simulink model "digitalIntegration"  (R2020a)
settings: Solver=FixedStepDiscrete  StartTime=0.0  StopTime=20  FixedStep=T  RelTol=1e-3
undefined symbols (not defined in the file): T
settings Model: Creator=mtcer  LastModifiedBy=mc218k
settings DataIOCC: ReturnWorkspaceOutputs=off
settings DebuggingCC: ArithmeticOperatorsInVariantConditions=warning
settings SFSimCC: CustomCodeUndefinedFunction=UseInterfaceOnly

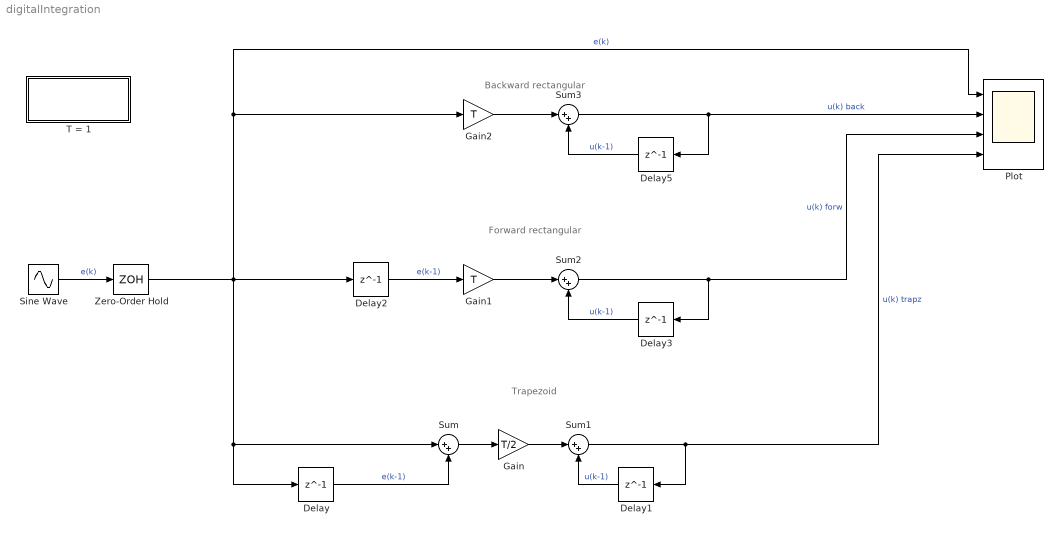
== system digitalIntegration ==
  note: Forward rectangular
  note: Trapezoid
  note: Backward rectangular
  Delay{,1..3,5} (5 alike) : Delay  DelayLength=1
  Gain : Gain  Gain=T/2
  Gain1 : Gain  Gain=T
  Gain2 : Gain  Gain=T
  Plot : Scope  NumInputPorts=4
  Sine Wave : Sin  SampleTime=0
  Sum{,1..3} (4 alike) : Sum  Inputs=|++
  T = 1 : Subsystem
      settings: OpenFcn=T=1;
  Zero-Order Hold : ZeroOrderHold  SampleTime=-1
  wires:
  Delay/1 -> Sum/2  "e(k-1)"
  Sum/1 -> Gain/1
  Gain/1 -> Sum1/1
  Sum1/1 -> Plot/4, Delay1/1  "u(k) trapz"
  Delay1/1 -> Sum1/2  "u(k-1)"
  Delay2/1 -> Gain1/1  "e(k-1)"
  Sum2/1 -> Plot/3, Delay3/1  "u(k) forw"
  Delay3/1 -> Sum2/2  "u(k-1)"
  Gain1/1 -> Sum2/1
  Gain2/1 -> Sum3/1
  Delay5/1 -> Sum3/2  "u(k-1)"
  Sum3/1 -> Delay5/1, Plot/2  "u(k) back"
  Sine Wave/1 -> Zero-Order Hold/1  "e(k)"
  Zero-Order Hold/1 -> Sum/1, Delay/1, Plot/1, Gain2/1, Delay2/1  "e(k)"

== system digitalIntegration/T = 1 ==
